simulink model "PVFCHEV_1"  (R2018a)
settings: Solver=VariableStepAuto  StartTime=0.0  StopTime=25  RelTol=1e-3
values from neighbouring files (symbols this model uses):
  Fc_current = [ 0  1.7  3.3  5.06  6.8   8.6  10.4   12.3  14.15   16   17.85  19.8   21.8   23.75   25.75   27.75  29.8  31.9  34.1  36.2  38.2  40.9  42.6  44.7   47.1   49.4   51.6    54   56.85  58.75  61.2  63.6  66.1  68.6  71.2  73.8 76.5 79.15  81.85  84.6  87.5   90.4  93.3      96.4   99.45  102.5    105.65   109   112.8  115.75  119.25   123     126.65     130.5      134.5   138.6  142.9 147.4  153.0 ...(+15 chars)    [pvfchev_configration.m]
  Fc_power = [ 0  100  200  300   400   500   600    700   800   900   1000   1100   1200   1300    1400    1500  1600   1700  1800  1900  2000  2100  2200  2300   2400   2500   2600   2700   2800  2900   3000  3100  3200 3300   3400  3500 3600 3700  3800   3900   4000   4100  4198.5    4300   4400   4500      4600   4700  4800    4900    5000    5100     5200       5300       5400    5500  5600  5700   5800   ...(+17 chars)    [pvfchev_configration.m]
  Ts_Control = 1e-04    (= 0.0001)    [pvfchev_configration.m]
  Ts_Power = 2e-06    [pvfchev_configration.m]
undefined symbols (not defined in the file or in its folder): DiscIntNeverNeededParam, Ion, Lithium
libraries: powerlib x30, powerlib_meascontrol x8, sdl_lib x8, fl_lib x6, nesl_utility x6, electricdrivelib x4, spsVIMeasurementModel x3, simulink x2, re_lib x1, spsDrivesPrivateModels x1, spsDrivesOutputSelector x1, spsDrivesSpeedControllerModel x1
(part 1 of 2)
settings Model: Creator=EUROPE LAPTOP  LastModifiedBy=Windows.10
settings SolverCC: AlgebraicLoopSolver=LineSearch
settings CodeAppCC: StateflowObjectComments=on
settings SimscapeCC: SimscapeNormalizeSystem=off

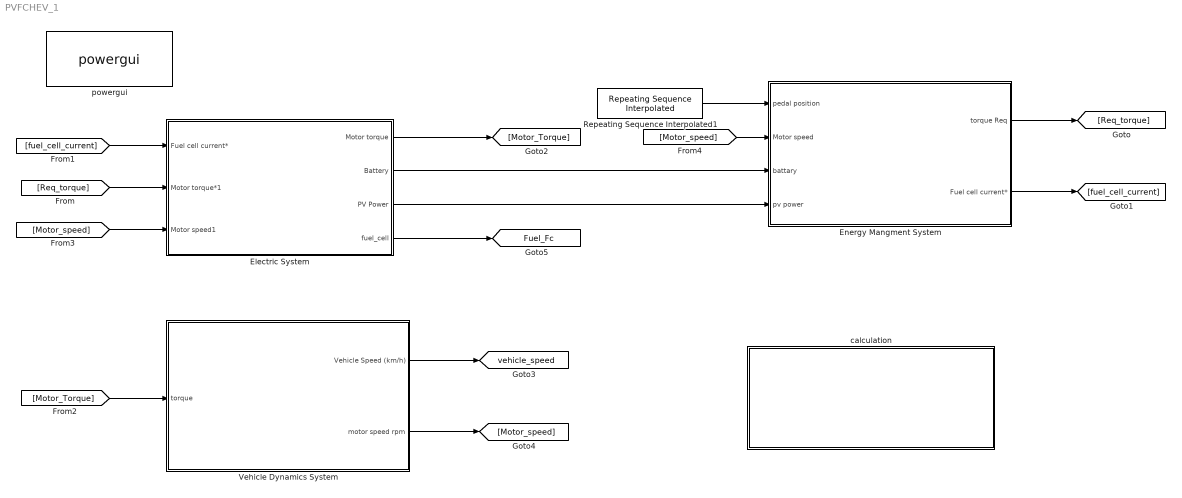
== system PVFCHEV_1 ==
  Electric System : Subsystem
  Energy Mangment System : Subsystem
  Repeating Sequence Interpolated1 : simulink/Sources/Repeating Sequence Interpolated  OutValues="[ 0 0 70 70 25 25  85  85 -70 -70].'"  TimeValues=[0 1.999 2 6 6.001 11 11.001 15.999 16 25].'  LookUpMeth=Interpolation-Use End Values  tsamp=0.01  OutMin=[]  OutMax=[]  OutDataTypeStr=double  OutputDataTypeScalingMode=double  OutDataType=fixdt(0,8)  OutScaling=2^-10
  Vehicle Dynamics System : Subsystem
  calculation : Subsystem
  powergui : powerlib/powergui  Priority=2  SimulationMode=Discrete  SampleTime=2e-6  frequency=60  Iterations=50  frequencyindice=0  Pbase=100e6  ErrMax=1e-4  UnitsV=kV  UnitsW=MW  buscounter=0  FunctionMessages=off  echomessages=off  EnableUseOfTLC=off  CurrentSourceSwitches=off  DisableSnubberDevices=off  DisableRonSwitches=off  DisableVfSwitches=off  DisplayEquations=off  SolverType=Tustin/Backward Euler (TBE)  Interpol=off  ExternalGateDelay=off  methode=off  Ts=100  x0status=blocks  SPID=off  SwTol=0  HookPort=off  RestoreLinks=warning  ResistiveCurrentMeasurement=off  Frange=[0:2:500]  Ylog=off  Xlog=on  ShowGrid=off  save=off  variable=ZData  structure=0  ZoomFFT=on  StartTime=0.0  cycles=1  DisplayStyle=1  fundamental=60  FreqAxis=off  MaxFrequency=1000  frequencyindicesteady=1  RmsSteady=1  display=off
  tag scope: Fuel_Fc=global, vehicle_speed=global
  wires:
  Energy Mangment System/2(Fuel cell current*) -> [fuel_cell_current]
  Electric System/1(Motor torque) -> [Motor_Torque]
  Electric System/3(PV Power) -> Energy Mangment System/4(pv power)
  [fuel_cell_current] -> Electric System/1("Fuel cell current* ")
  [Motor_Torque] -> Vehicle Dynamics System/1(torque)
  [Req_torque] -> Electric System/2(Motor torque*1)
  [Motor_speed] -> Energy Mangment System/2(Motor speed)
  Repeating Sequence Interpolated1/1 -> Energy Mangment System/1(pedal position)
  Energy Mangment System/1("torque Req ") -> [Req_torque]
  Vehicle Dynamics System/1(Vehicle Speed (km/h)) -> [vehicle_speed]
  Vehicle Dynamics System/2(motor speed rpm) -> [Motor_speed]
  [Motor_speed] -> Electric System/3(Motor speed1)
  Electric System/2(Battery) -> Energy Mangment System/3(battary)
  Electric System/4(fuel_cell) -> [Fuel_Fc]

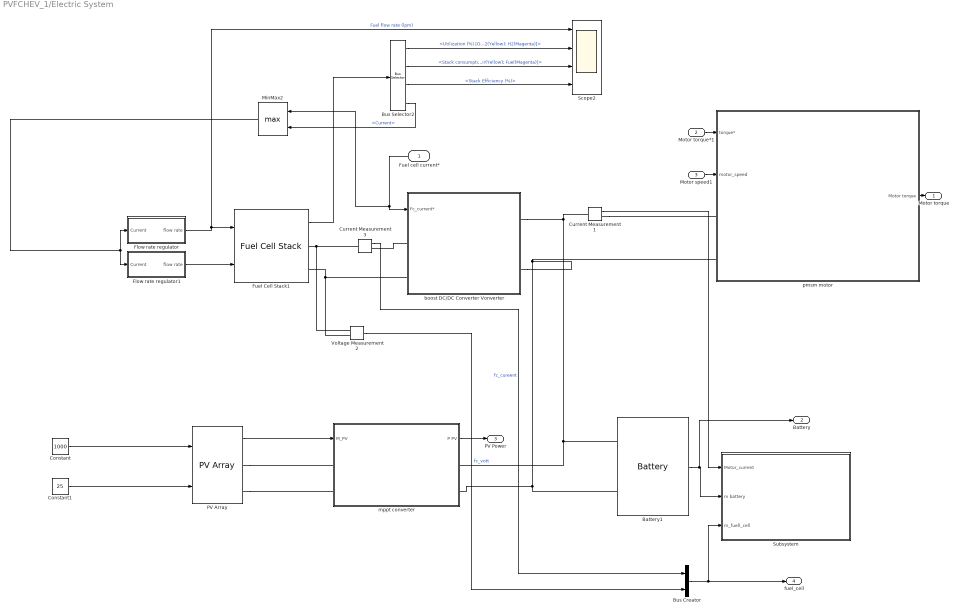
== system PVFCHEV_1/Electric System ==
  "Fuel cell current* " : Inport
  Motor torque*1 : Inport  Port=2
  Motor speed1 : Inport  Port=3
  Battery1 : electricdrivelib/Extra Sources/Battery  BatType=Lithium-Ion  ShowTempParam=off  ThermalPreset=no  ShowAgeParam=off  NomV=144  NomQ=9.6  SOC=74  Batt_Tr=30  PresetModel=on  MaxQ=9.6  MinV=108  FullV=167.6141  Dis_rate=4.1739  R=0.15  Normal_OP=8.6817  expZone="[155.5756     0.4716522]"  current=[6.5 13 32.5]  Units=Time  Tci=20  NomT=20  T2=-30  MaxQ2=4.8  FullV2=7.1  Normal_OP2=5.655  expZone2="[6.58           1]"  Rca=0.6  ti=2000  Dp=0  Neq0=0  Tsim=1e6  Ta1=25  Qeol=5.4*0.9  Reol=0.013333*1.2  Char_age=[2.3478, 3]  Dis_age=[2.3478, 10]  N1=1500  N2=10500  N3=1000  N4=1400  Ta2=45  N5=950
  Bus Creator : BusCreator  Inputs=2
  Bus Selector2 : BusSelector  OutputSignals=Utilization (%) [O2(Yellow); H2(Magenta)],Stack consumption (lpm) [Air(Yellow); Fuel(Magenta)],Stack Efficiency (%),Current
  Constant : Constant  Value=1000
  Constant1 : Constant  Value=25
  Current Measurement1 : powerlib/Measurements/Current Measurement  PhasorSimulation=off  OutputType=Complex  PSBequivalent=0
  Current Measurement3 : powerlib/Measurements/Current Measurement  PhasorSimulation=off  OutputType=Complex  PSBequivalent=0
  Flow rate regulator : Subsystem  mask{Nc=65, Uf_H2=99.56, T=65, Pf=1.5, x=99.95}
      mask prompts: Nc "Number of cells"; Uf_H2 "Nominal Hydrogen utilization (%)"; T "Operating temperature (Celsius)"; Pf "Fuel pressure (bar)"; x "H2 composition (%)"
  Flow rate regulator1 : Subsystem  mask{Nc=65, Uf_H2=99.56, T=65, Pf=1.5, x=99.95}
      mask prompts: Nc "Number of cells"; Uf_H2 "Nominal Hydrogen utilization (%)"; T "Operating temperature (Celsius)"; Pf "Fuel pressure (bar)"; x "H2 composition (%)"
  Fuel Cell Stack1 : electricdrivelib/Extra Sources/Fuel Cell Stack  PresetModel=No (User-Defined)  FcType=Proton Exchange Membrane (PEM)  Detailed=Detailed  Eoc="[65  63]"  NomVI="[93.3            45]"  EndVI="[162.16   37]"  Nc=65  n=55  TOp=65  AirFr=300  SuppPress="[1.5           1]"  Comp="[99.95           21            1]"  SignX=off  SignY=off  FlowRateH2=on  FlowRateAir=on  SystemTemp=off  SystemPH2=off  SystemPAir=off  FCDyn=off  FC_tau=0  Peak_O2=80  V_Under=10
      settings: SourceProductName=Simscape Power Systems  SourceProductBaseCode=PS
  MinMax2 : MinMax  Function=max  Inputs=2
  PV Array : re_lib/Solar/PV Array  Npar=1  Nser=2  PlotType=array @ 1000 W/m2 & specified temperatures  S_vec="[ 1000  500  100 ]"  Temp_C_vec="[  25  ]"  ModuleName=User-defined  PlotWhenSelected=off  Pm=249.952  Ncell=72  Voc=50.93  Isc=6.2  Vm=42.8  Im=5.84  beta_Voc_pc=-0.36099  alpha_Isc_pc=0.102  beta_Voc=-0.18385  alpha_Isc=0.006324  IL=6.2189  I0=2.3129e-10  nI=1.1472  Rsh=540.4905  Rs=0.29328  BAL=on  Tc=1e-6  Tfilter=5e-5
  Scope2 : Scope  NumInputPorts=4
  Subsystem : Subsystem
  Voltage Measurement2 : powerlib/Measurements/Voltage Measurement  PhasorSimulation=off  OutputType=Complex  PSBequivalent=0
  boost DC/DC Converter Vonverter : Subsystem
  mppt converter : Subsystem
  pmsm motor : Subsystem
      mask Display: image('C:\Users\Windows.10\Desktop\motor.png');
  Motor torque : Outport
  Battery : Outport  Port=2
  PV Power : Outport  Port=3
  fuel_cell : Outport  Port=4
  wires:
  pmsm motor/1(Motor torque) -> Motor torque/1
  Constant/1 -> PV Array/1
  Constant1/1 -> PV Array/2
  Bus Selector2/1 -> Scope2/2  "<Utilization (%) [O2(Yellow); H2(Magenta)]>"
  Bus Selector2/2 -> Scope2/3  "<Stack consumption (lpm) [Air(Yellow); Fuel(Magenta)]>"
  Fuel Cell Stack1/1 -> Bus Selector2/1
  Flow rate regulator/1(flow rate) -> Fuel Cell Stack1/1, Scope2/1  "Fuel flow rate (lpm)"
  MinMax2/1 -> Flow rate regulator/1(Current), Flow rate regulator1/1(Current)
  Flow rate regulator1/1(flow rate) -> Fuel Cell Stack1/2
  "Fuel cell current* "/1 -> MinMax2/1, boost DC/DC Converter Vonverter/1(Fc_current*)
  Current Measurement3/1 -> Bus Creator/1  "fc_cureent"
  Bus Selector2/3 -> Scope2/4  "<Stack Efficiency (%)>"
  Voltage Measurement2/1 -> Bus Creator/2  "fc_vott"
  Motor speed1/1 -> pmsm motor/2(motor_speed)
  Motor torque*1/1 -> pmsm motor/1(torque*)
  Battery1/1 -> Subsystem/2(m battery), Battery/1
  PV Array/1 -> mppt converter/1(M_PV)
  mppt converter/1(P PV) -> PV Power/1
  Bus Creator/1 -> Subsystem/3(m_fuell_cell), fuel_cell/1
  Current Measurement1/1 -> Subsystem/1(Motor_current)
  Bus Selector2/4 -> MinMax2/2  "<Current>"
  connections:
  PV Array/RConn1 -- mppt converter/LConn1
  PV Array/RConn2 -- mppt converter/LConn2
  Battery1/LConn1 -- mppt converter/RConn1 -- Current Measurement1/LConn1 -- boost DC/DC Converter Vonverter/RConn1
  Current Measurement3/LConn1 -- Voltage Measurement2/LConn1 -- Fuel Cell Stack1/RConn1
  boost DC/DC Converter Vonverter/LConn1 -- Current Measurement3/RConn1
  Voltage Measurement2/LConn2 -- Fuel Cell Stack1/RConn2 -- boost DC/DC Converter Vonverter/LConn2
  pmsm motor/LConn2 -- boost DC/DC Converter Vonverter/RConn2 -- mppt converter/RConn2 -- Battery1/LConn2
  Current Measurement1/RConn1 -- pmsm motor/LConn1

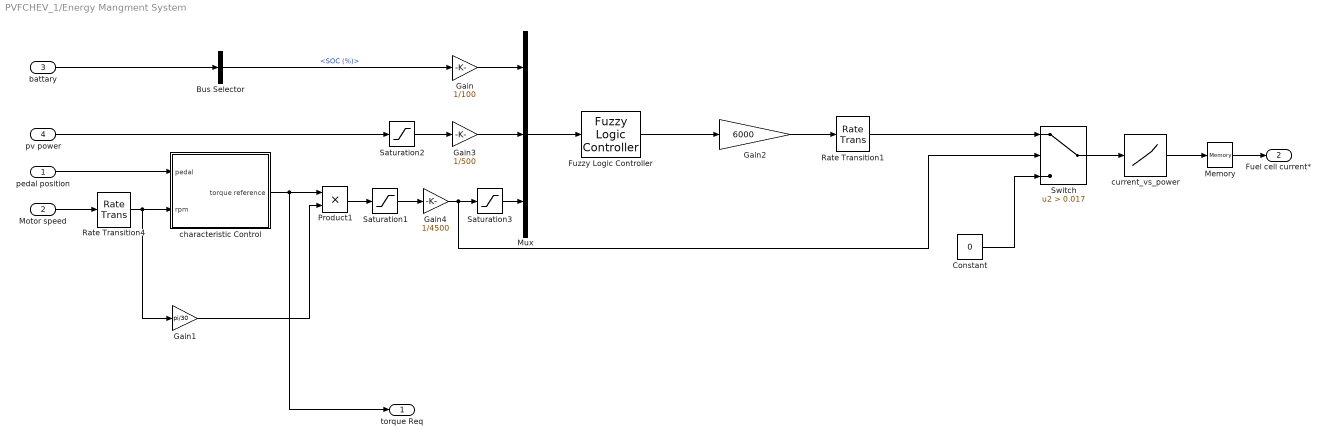
== system PVFCHEV_1/Energy Mangment System ==
  pedal position : Inport
  Motor speed : Inport  Port=2
  battary : Inport  Port=3
  pv power : Inport  Port=4
  Bus Selector : BusSelector  OutputSignals=SOC (%)
  Constant : Constant  Value=0
  Fuzzy Logic Controller : fuzblock/Fuzzy Logic  Controller  FIS=power_mangment  OutputSampleNumber=101  DataType=double  FuzzifiedInputs=off  RuleFiringStrengths=off  RuleOutputs=off  AggregatedOutputs=off  SimulateUsing=Interpreted execution  OutOfRangeInputValueMessage=warning  NoRuleFiredMessage=warning  EmptyOutputFuzzySetMessage=warning
  Gain : Gain  Gain=1/100
  Gain1 : Gain  Gain=pi/30
  Gain2 : Gain  Gain=6000
  Gain3 : Gain  Gain=1/500
  Gain4 : Gain  Gain=1/4500
  Memory : Memory  InitialCondition=0.00001
  Mux : Mux  Inputs=3
  Product1 : Product
  Rate Transition1 : RateTransition
  Rate Transition4 : RateTransition
  Saturation1 : Saturate  UpperLimit=4500  LowerLimit=-5000
  Saturation2 : Saturate  UpperLimit=500  LowerLimit=0
  Saturation3 : Saturate  UpperLimit=1  LowerLimit=0
  Switch : Switch  Criteria=u2 > Threshold  Threshold=0.017
  characteristic Control : Subsystem
  current_vs_power : Lookup  InputValues=Fc_power  Table=Fc_current
  "torque Req " : Outport
  Fuel cell current* : Outport  Port=2
  wires:
  battary/1 -> Bus Selector/1
  Bus Selector/1 -> Gain/1  "<SOC (%)>"
  pedal position/1 -> characteristic Control/1(pedal)
  Motor speed/1 -> Rate Transition4/1
  characteristic Control/1(torque reference) -> "torque Req "/1, Product1/1
  Mux/1 -> Fuzzy Logic Controller/1
  Fuzzy Logic Controller/1 -> Gain2/1
  Gain/1 -> Mux/1
  pv power/1 -> Saturation2/1
  Gain3/1 -> Mux/2
  Gain4/1 -> Saturation3/1, Switch/2
  Saturation2/1 -> Gain3/1
  Saturation1/1 -> Gain4/1
  current_vs_power/1 -> Memory/1
  Rate Transition4/1 -> Gain1/1, characteristic Control/2(rpm)
  Product1/1 -> Saturation1/1
  Gain2/1 -> Rate Transition1/1
  Constant/1 -> Switch/3
  Switch/1 -> current_vs_power/1
  Rate Transition1/1 -> Switch/1
  Memory/1 -> Fuel cell current*/1
  Gain1/1 -> Product1/2
  Saturation3/1 -> Mux/3

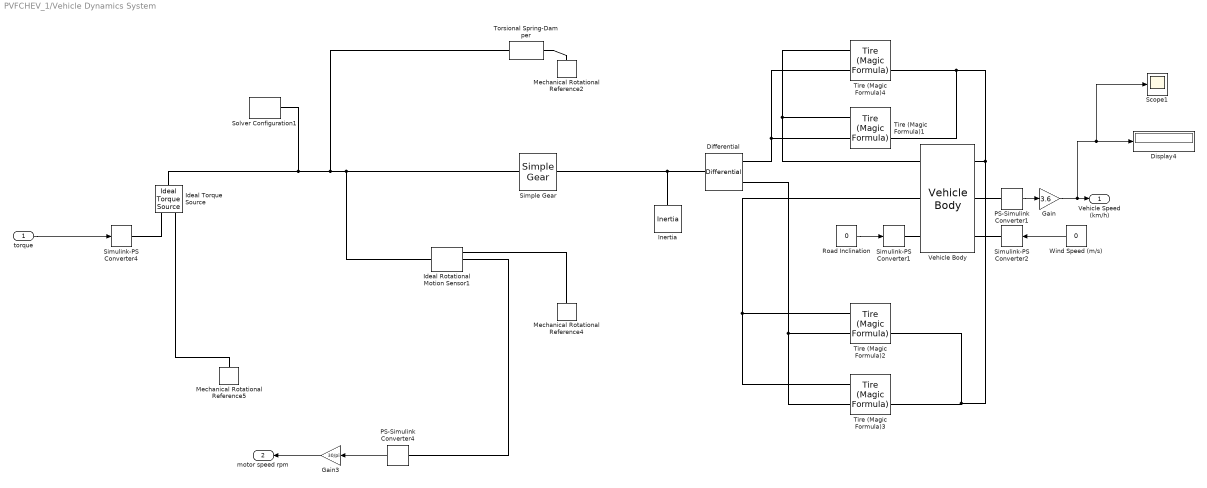
== system PVFCHEV_1/Vehicle Dynamics System ==
  torque : Inport
  Differential : sdl_lib/Gears/Differential  driveshaft_location=2  cd_ratio=1.2  friction_model=1  efficiency=[ 0.85 0.92 ]  mu_visc=[ 0 0 ] N*m/(rad/s)  pwr_thr=[ 0.001 0.001 ] W  carrier_inertia=0.001 kg*m^2  planet_inertia=0.0001 kg*m^2  temperature_TLU=[ 280 300 320 ] K  efficiency_ss_TLU=[ 0.95 0.9 0.85 ]  efficiency_cd_TLU=[ 0.95 0.9 0.85 ]  thermal_mass=50 J/K  T_init=300 K
      settings: SourceProductName=Simscape Driveline  SourceProductBaseCode=LD
  Display4 : Display
  Gain : Gain  Gain=3.6
  Gain3 : Gain  Gain=30/pi
  Ideal Rotational Motion Sensor1 : fl_lib/Mechanical/Mechanical Sensors/Ideal Rotational Motion Sensor  offset=0 rad
  Ideal Torque Source : fl_lib/Mechanical/Mechanical Sources/Ideal Torque Source
  Inertia : fl_lib/Mechanical/Rotational Elements/Inertia  inertia=0.0000001 kg*m^2  w_specify=off  w_priority=High  w=0 rad/s  w_nominal_specify=off  w_nominal_unit=rad/s  w_nominal_value=1  t_specify=off  t_priority=None  t=0 N*m  t_nominal_specify=off  t_nominal_unit=N*m  t_nominal_value=1
  Mechanical Rotational Reference2 : fl_lib/Mechanical/Rotational Elements/Mechanical Rotational Reference
  Mechanical Rotational Reference4 : fl_lib/Mechanical/Rotational Elements/Mechanical Rotational Reference
  Mechanical Rotational Reference5 : fl_lib/Mechanical/Rotational Elements/Mechanical Rotational Reference
  PS-Simulink Converter1 : nesl_utility/PS-Simulink Converter  PhysicalDomain=network_engine_domain  SubClassName=ps_output  LeftPortType=input  RightPortType=output  PseudoPeriodic=off  Frequencies=[]  Unit=m/s  AffineConversion=off
  PS-Simulink Converter4 : nesl_utility/PS-Simulink Converter  PhysicalDomain=network_engine_domain  SubClassName=ps_output  LeftPortType=input  RightPortType=output  PseudoPeriodic=off  Frequencies=[]  Unit=rad/s  AffineConversion=off
  Road Inclination : Constant  Value=0
  Scope1 : Scope
  Simple Gear : sdl_lib/Gears/Simple Gear  ratio=3  rotation_direction=1  friction_model=1  T_noload=0.1 N*m  T_nom=5 N*m  efficiency_nom=0.8  efficiency=0.8  mu_visc=[ 0 0 ] N*m/(rad/s)  w_thr=0.01 rad/s  pwr_thr=0.001 W  temperature_TLU=[ 280 300 320 ] K  load_TLU=[ 1 5 10 ] N*m  efficiency_TLU=[ 0.95 0.9 0.85 ]  efficiency_TLU2=[ 0.85 0.8 0.75; 0.95 0.9 0.85; 0.85 0.8 0.7 ]  thermal_mass=50 J/K  T_init=300 K
      settings: SourceProductName=Simscape Driveline
  Simulink-PS Converter1 : nesl_utility/Simulink-PS Converter  PhysicalDomain=network_engine_domain  SubClassName=ps_input  LeftPortType=input  RightPortType=output  PseudoPeriodic=off  Frequencies=[]  NoiseDistribution=none  NoiseParameters=[]  Unit=rad  AffineConversion=off  FilteringAndDerivatives=zero  SimscapeFilterOrder=1  InputFilterTimeConstant=.001  UdotUserProvided=1
  Simulink-PS Converter2 : nesl_utility/Simulink-PS Converter  PhysicalDomain=network_engine_domain  SubClassName=ps_input  LeftPortType=input  RightPortType=output  PseudoPeriodic=off  Frequencies=[]  NoiseDistribution=none  NoiseParameters=[]  Unit=m/s  AffineConversion=off  FilteringAndDerivatives=zero  SimscapeFilterOrder=1  InputFilterTimeConstant=.001  UdotUserProvided=1
  Simulink-PS Converter4 : nesl_utility/Simulink-PS Converter  PhysicalDomain=network_engine_domain  SubClassName=ps_input  LeftPortType=input  RightPortType=output  PseudoPeriodic=off  Frequencies=[]  NoiseDistribution=none  NoiseParameters=[]  Unit=N*m  AffineConversion=off  FilteringAndDerivatives=zero  SimscapeFilterOrder=1  InputFilterTimeConstant=.001  UdotUserProvided=1
  Solver Configuration1 : nesl_utility/Solver Configuration  PhysicalDomain=network_engine_domain  SubClassName=solver  LeftPortType=input  RightPortType=generic  Tones=[]  Harmonics=[]  SimulateNoise=off  Profile=off  UseLocalSampling=off  EnableSwitchedLinearOptims=on  FrequencyDomain=off  UseCCode=off  RelTol=0.001  AbsTol=1e-06  MinStep=1e-09  ToWorkspace=off  RevertToSquareIcSolve=off  NumHomotopyIterations=100  PhasorMode=off  PhasorModeNumHarmonics=1  DoDC=off  ResidualTolerance=1e-9  UseLocalSolver=on  LocalSolverChoice=NE_BACKWARD_EULER_ADVANCER  LocalSolverSampleTime=.001  DoFixedCost=on  MaxNonlinIter=3  MaxModeIter=2  LinearAlgebra=Sparse  EquationFormulation=NE_TIME_EF  DelaysMemoryBudget=1024  AutomaticFiltering=on  FilteringTimeConstant=0.001
  Tire (Magic Formula){1..4} (4 alike) : sdl_lib/Tires & Vehicles/Tire (Magic Formula)  parameterization=3  F_z1=1e+3 N  F_x1=3.5e+3 N  kappa1=10  B_m=10  C_m=1.9  D_m=1  E_m=0.97  fz0=4e+3 N  p_Cx=1.685  p_Dx=[ 1.21 -0.037 ]  p_Ex=[ 0.344 0.095 -0.02 0 ]  p_Kx=[ 21.51 -0.163 0.245 ]  p_Hx=[ -0.002 0.002 ]  p_Vx=[ 0 0 ]  v_tr_thr=0.1 m/s  r_e=0.2 m  model_compliance=0  stiffness=1e+6 N/m  damping=1000 N/(m/s)  model_inertia=0  inertia=1 kg*m^2  initial_velocity=0 rad/s  model_resistance=0  resistance_model=1  coeff=0.015  p_tire=250e3 Pa  alpha=-0.003  beta=0.97  coeff_a=84e-4  coeff_b=6.2e-4 s/m  coeff_c=1.6e-4 s^2/m^2  v_thr=1e-3 m/s
      settings: SourceProductName=Simscape Driveline
  Torsional Spring-Damper : sdl_lib/Couplings & Drives/Torsional Spring-Damper  k=0.0000005 N*m/rad  mu_visc=0.0000003 N*m/(rad/s)  trq_coulomb=0 N*m  static_kinetic_ratio=1.1  w_tol=0.001 rad/s  model_hardstop=0  upper_bound=10 deg  lower_bound=-10 deg  k_endstop=1e+6 N*m/rad  D_endstop=10 N*m/(rad/s)  hardstop_model=3  transition=0.001 rad  x0=0 deg
      settings: SourceProductName=Simscape Driveline  SourceProductBaseCode=LD
  Vehicle Body : sdl_lib/Tires & Vehicles/Vehicle Body  mass=800 kg  n_w=2  x_f=1 m  x_r=0.35 m  y_c=0.7 m  model_pitch=0  inertia=4000 kg*m^2  suspension_model=1  k_f=1e4 N/m  b_f=1e4 N/(m/s)  k_r=1e4 N/m  b_r=1e4 N/(m/s)  k_f_TLU=[-2000, -1000, 0, 1000, 2000] N  x_f_TLU=[-.4, -.2, 0, .2, .4] m  b_f_TLU=[-200, -100, 0, 100, 200] N  v_f_TLU=[-4, -2, 0, 2, 4] m/s  k_r_TLU=[-2000, -1000, 0, 1000, 2000] N  x_r_TLU=[-.4, -.2, 0, .2, .4] m  b_r_TLU=[-200, -100, 0, 100, 200] N  v_r_TLU=[-4, -2, 0, 2, 4] m/s  interp_method=simscape.enum.interpolation.linear  extrap_method=simscape.enum.extrapolation.linear  model_hardstop=0  upper_bound_f=.25 m  lower_bound_f=-.25 m  stop_k_f=1e6 N/m  stop_b_f=150 N/(m/s)  upper_bound_r=.25 m  lower_bound_r=-.25 m  stop_k_r=1e6 N/m  stop_b_r=150 N/(m/s)  initial_pitch=0 rad  initial_pitch_rate=0 rad/s  g=9.81 m/s^2  liftoff_warning=0  area=2.3 m^2  Cd=0.36  rho=1.18 kg/m^3  v_specify=on  v_priority=High  v=0 m/s  v_nominal_specify=off  v_nominal_unit=m/s  v_nominal_value=1
      settings: SourceProductName=Simscape Driveline
  Wind Speed (m/s) : Constant  Value=0
  Vehicle Speed (km/h) : Outport
  motor speed rpm : Outport  Port=2
  wires:
  Gain3/1 -> motor speed rpm/1
  torque/1 -> Simulink-PS Converter4/1
  PS-Simulink Converter1/1 -> Gain/1
  Wind Speed (m/s)/1 -> Simulink-PS Converter2/1
  Road Inclination/1 -> Simulink-PS Converter1/1
  PS-Simulink Converter4/1 -> Gain3/1
  Gain/1 -> Scope1/1, Display4/1, Vehicle Speed (km/h)/1
  connections:
  Tire (Magic Formula)2/LConn1 -- Vehicle Body/RConn2 -- Tire (Magic Formula)3/LConn1
  Tire (Magic Formula)2/RConn2 -- Vehicle Body/LConn1 -- Tire (Magic Formula)1/RConn2 -- Tire (Magic Formula)4/RConn2 -- Tire (Magic Formula)3/RConn2
  Tire (Magic Formula)2/LConn2 -- Tire (Magic Formula)3/LConn2 -- Differential/RConn1
  Tire (Magic Formula)1/LConn2 -- Tire (Magic Formula)4/LConn2 -- Differential/RConn2
  Tire (Magic Formula)4/LConn1 -- Vehicle Body/RConn1 -- Tire (Magic Formula)1/LConn1
  Differential/LConn1 -- Inertia/LConn1 -- Simple Gear/RConn1
  Mechanical Rotational Reference4/LConn1 -- Ideal Rotational Motion Sensor1/RConn1
  Simulink-PS Converter2/RConn1 -- Vehicle Body/LConn3
  Ideal Rotational Motion Sensor1/RConn2 -- PS-Simulink Converter4/LConn1
  Ideal Torque Source/LConn1 -- Solver Configuration1/RConn1 -- Torsional Spring-Damper/LConn1 -- Ideal Rotational Motion Sensor1/LConn1 -- Simple Gear/LConn1
  Torsional Spring-Damper/RConn1 -- Mechanical Rotational Reference2/LConn1
  Mechanical Rotational Reference5/LConn1 -- Ideal Torque Source/RConn2
  Simulink-PS Converter1/RConn1 -- Vehicle Body/RConn3
  PS-Simulink Converter1/LConn1 -- Vehicle Body/LConn2
  Simulink-PS Converter4/RConn1 -- Ideal Torque Source/RConn1

== system PVFCHEV_1/calculation ==
  Add2 : Sum  Inputs=+++-
  Mux2 : Mux  Inputs=6
  To File1 : ToFile  Filename=power.mat  MatrixName=power
  power_balance : Scope
  power_distrbution : Scope
  wires:
  [mot_power_Ts] -> Add2/4
  [bat_power_Ts] -> Add2/2
  [fc_power_out_Ts] -> Add2/1
  [pv_power_Ts] -> Add2/3
  Add2/1 -> power_balance/1
  [bat_power_Ts] -> Mux2/1  "bat"
  [fc_power_out_Ts] -> Mux2/2  "fc"
  [pv_power_Ts] -> Mux2/3  "pv"
  [mot_power_Ts] -> Mux2/4  "mot"
  [pv_power_source] -> Mux2/5  "pv_source"
  [fc_power_source] -> Mux2/6  "fc_source"
  Mux2/1 -> power_distrbution/1, To File1/1

== system PVFCHEV_1/Electric System/Flow rate regulator ==
  Current : Inport
  Fcn1 : Fcn  Expr=60000*8.3145*(273+T)*Nc*u(1)/(2*96485*(Pf*101325)*Uf_H2/100*x/100)
  Saturation : Saturate  UpperLimit=inf  LowerLimit=1
  flow rate : Outport
  wires:
  Fcn1/1 -> Saturation/1
  Current/1 -> Fcn1/1
  Saturation/1 -> flow rate/1

== system PVFCHEV_1/Electric System/Flow rate regulator1 ==
  Current : Inport
  Fcn1 : Fcn  Expr=60000*8.3145*(273+T)*65*u(1)/(4*96485*(0.9*101325)*0.5057*0.21)
  Saturation : Saturate  UpperLimit=inf  LowerLimit=1
  flow rate : Outport
  wires:
  Saturation/1 -> flow rate/1
  Current/1 -> Fcn1/1
  Fcn1/1 -> Saturation/1

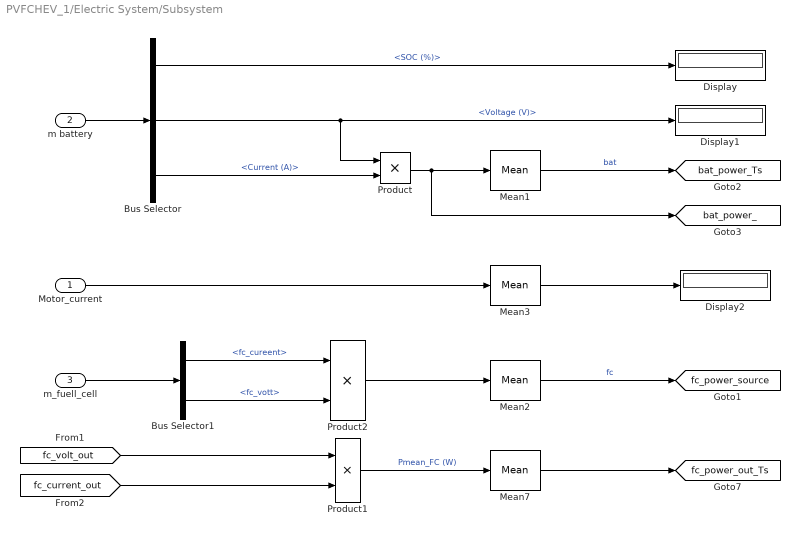
== system PVFCHEV_1/Electric System/Subsystem ==
  Motor_current : Inport
  m battery : Inport  Port=2
  m_fuell_cell : Inport  Port=3
  Bus Selector : BusSelector  OutputSignals=SOC (%),Voltage (V),Current (A)
  Bus Selector1 : BusSelector  OutputSignals=fc_cureent,fc_vott
  Display : Display
  Display1 : Display
  Display2 : Display
  Mean{1..3,7} (4 alike) : powerlib_meascontrol/Measurements/Mean  Freq=60  Vinit=0  Ts=Ts_Control
  Product : Product
  Product1 : Product  RndMeth=Zero
  Product2 : Product  RndMeth=Zero
  tag scope: bat_power_=global, bat_power_Ts=global, fc_power_out_Ts=global, fc_power_source=global
  wires:
  m battery/1 -> Bus Selector/1
  Bus Selector/1 -> Display/1  "<SOC (%)>"
  Bus Selector/2 -> Product/1, Display1/1  "<Voltage (V)>"
  Bus Selector/3 -> Product/2  "<Current (A)>"
  Motor_current/1 -> Mean3/1
  m_fuell_cell/1 -> Bus Selector1/1
  Product1/1 -> Mean7/1  "Pmean_FC (W)"
  Product/1 -> Mean1/1, [bat_power_]
  Bus Selector1/1 -> Product2/1  "<fc_cureent>"
  Bus Selector1/2 -> Product2/2  "<fc_vott>"
  [fc_volt_out] -> Product1/1
  [fc_current_out] -> Product1/2
  Mean1/1 -> [bat_power_Ts]  "bat"
  Product2/1 -> Mean2/1
  Mean2/1 -> [fc_power_source]  "fc"
  Mean3/1 -> Display2/1
  Mean7/1 -> [fc_power_out_Ts]

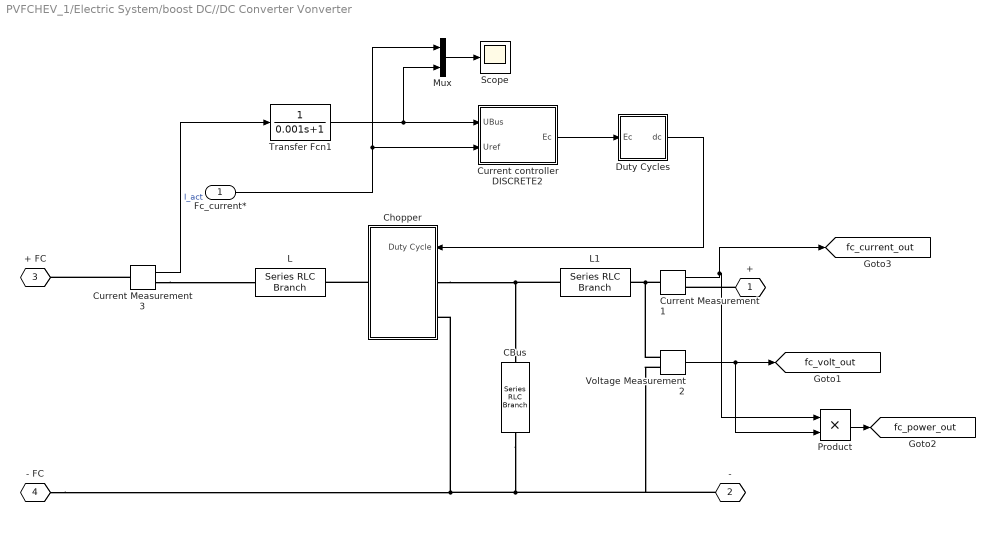
== system PVFCHEV_1/Electric System/boost DC//DC Converter Vonverter ==
  Fc_current* : Inport
  CBus : powerlib/Elements/Series RLC Branch  LConnTagsString=__new0  RConnTagsString=__new0  BranchType=RC  Resistance=0.2  Inductance=1e-3  SetiL0=off  InitialCurrent=0  Capacitance=7500e-6  Setx0=on  InitialVoltage=152  Measurements=None
  Chopper : Subsystem  mask(SPSdrives Converter){SnubberResistance=10e3, SnubberCapacitance=inf, Ron=1e-3, ForwardVoltages=[1.3,1.3], IGBTParameters=[0,0], converterType=Inverter}
      mask prompts: SnubberResistance "Snubber resistance Rs (Ohms):"; SnubberCapacitance "Snubber capacitance Cs (F):"; Ron "Ron (Ohms):"; ForwardVoltages "Forward voltages [Device Vf(V), Diode Vd (V)]"; IGBTParameters "[Tf(s), Tt(s)]:"; converterType "Converter type:"
      mask help: This model implements an average-value buck converter."Duty Cycle" contains the duty cycle of the internal IGBT device.
      mask TypeOptions converterType: Rectifier | Inverter
      mask Display: plot(0,0,100,100,[39 39 23.8],[71 28 28],[44 56 49.6 56 52.8 56 61 61],[39.2 33.6 32.8 33.6 40.8 33.6 30 12.4],[44 44 44 61 61],[28 71 60 66.4 90],[75 67 83 75 67 83 75 75],[54 42 42 54 54 54 54 66],[61 75 75],[24 24 42],[75 75 61],[66,76,76])
  Current Measurement1 : powerlib/Measurements/Current Measurement  PhasorSimulation=off  OutputType=Complex  PSBequivalent=0
  Current Measurement3 : powerlib/Measurements/Current Measurement  PhasorSimulation=off  OutputType=Complex  PSBequivalent=0
  Current controller DISCRETE2 : Subsystem  mask(PI controller){Kp=0.0005, Ki=0.15, Ts=1e-3}
      mask prompts: Kp "Proportional gain (Kp)"; Ki "Integral gain (Ki)"; Ts "Sample time (s) :"
      mask help: Proportional-Integral Speed Controller
      mask Display: plot(0,0,100,100,[35,35,65],[70,30,30],[35,65],[45,60])
  Duty Cycles : Subsystem
  L : powerlib/Elements/Series RLC Branch  LConnTagsString=__new0  RConnTagsString=__new0  BranchType=L  Resistance=0.3  Inductance=500e-6  SetiL0=on  InitialCurrent=5  Capacitance=100e-6  Setx0=off  InitialVoltage=0  Measurements=None
  L1 : powerlib/Elements/Series RLC Branch  LConnTagsString=__new0  RConnTagsString=__new0  BranchType=L  Resistance=0.3  Inductance=500e-6  SetiL0=on  InitialCurrent=0.0001  Capacitance=100e-6  Setx0=off  InitialVoltage=0  Measurements=None
  Mux : Mux  Inputs=2
  Product : Product
  Scope : Scope
  Transfer Fcn1 : TransferFcn  Denominator=[0.001 1]
  Voltage Measurement2 : powerlib/Measurements/Voltage Measurement  PhasorSimulation=off  OutputType=Complex  PSBequivalent=0
  + : PMIOPort  Tag=PMCPort  Side=Right
  - : PMIOPort  Tag=PMCPort  Port=2  Side=Right
  + FC : PMIOPort  Tag=PMCPort  Port=3  Side=Left
  - FC : PMIOPort  Tag=PMCPort  Port=4  Side=Left
  tag scope: fc_current_out=global, fc_power_out=global, fc_volt_out=global
  wires:
  Duty Cycles/1(dc) -> Chopper/1(Duty Cycle)
  Current controller DISCRETE2/1(Ec) -> Duty Cycles/1(Ec)
  Fc_current*/1 -> Mux/1, Current controller DISCRETE2/2(Uref)
  Mux/1 -> Scope/1
  Current Measurement3/1 -> Transfer Fcn1/1  "I_act"
  Transfer Fcn1/1 -> Mux/2, Current controller DISCRETE2/1(UBus)
  Voltage Measurement2/1 -> Product/2, [fc_volt_out]
  Current Measurement1/1 -> Product/1, [fc_current_out]
  Product/1 -> [fc_power_out]
  connections:
  - FC/RConn1 -- -/RConn1 -- Voltage Measurement2/LConn2 -- CBus/RConn1 -- Chopper/LConn2
  Chopper/LConn1 -- L1/RConn1 -- CBus/LConn1
  Chopper/RConn1 -- L/LConn1
  Current Measurement3/LConn1 -- + FC/RConn1
  Current Measurement3/RConn1 -- L/RConn1
  Current Measurement1/LConn1 -- Voltage Measurement2/LConn1 -- L1/LConn1
  +/RConn1 -- Current Measurement1/RConn1

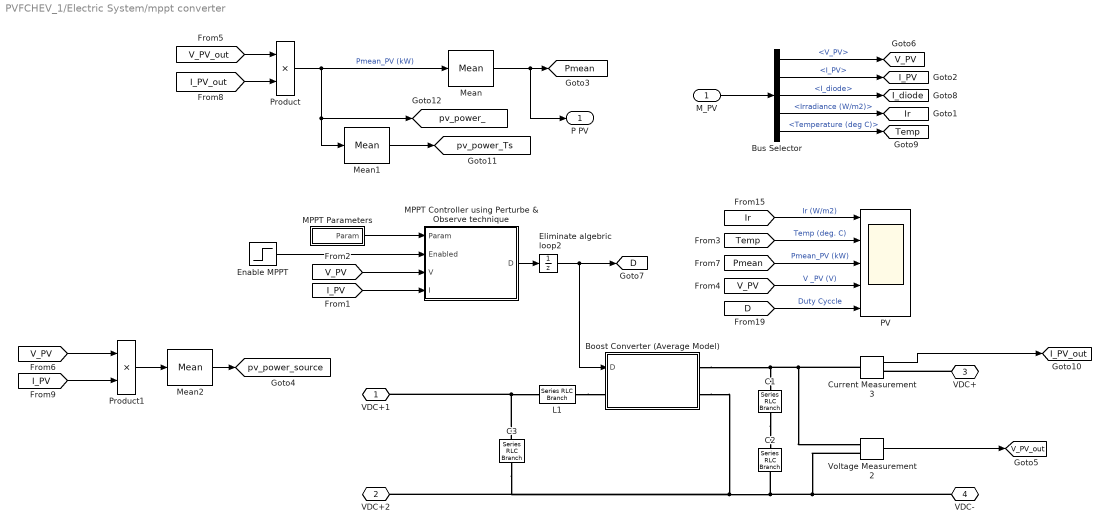
== system PVFCHEV_1/Electric System/mppt converter ==
  M_PV : Inport
  Boost Converter (Average Model) : Subsystem  mask(Boost Converter (Average Model)){Ts=Ts_Power}
      mask prompts: Ts "Sample time:"
      mask Display: disp('Boost\n(Average)')
  Bus Selector : BusSelector  OutputSignals=V_PV,I_PV,I_diode,Irradiance (W/m2),Temperature (deg C)
  C1 : powerlib/Elements/Series RLC Branch  LConnTagsString=__new0  RConnTagsString=__new0  BranchType=C  Resistance=1.0  Inductance=1.0  SetiL0=off  InitialCurrent=0  Capacitance=12000e-06  Setx0=off  InitialVoltage=0  Measurements=None
  C2 : powerlib/Elements/Series RLC Branch  LConnTagsString=__new0  RConnTagsString=__new0  BranchType=C  Resistance=1.0  Inductance=1.0  SetiL0=off  InitialCurrent=0  Capacitance=12000e-06  Setx0=off  InitialVoltage=0  Measurements=None
  C3 : powerlib/Elements/Series RLC Branch  LConnTagsString=__new0  RConnTagsString=__new0  BranchType=C  Resistance=1.0  Inductance=1.0  SetiL0=off  InitialCurrent=0  Capacitance=100e-6  Setx0=off  InitialVoltage=0  Measurements=Branch voltage
  Current Measurement3 : powerlib/Measurements/Current Measurement  PhasorSimulation=off  OutputType=Complex  PSBequivalent=0
  Eliminate algebric loop2 : UnitDelay  SampleTime=Ts_Control
  Enable MPPT : Step  Time=0.3  SampleTime=0
  L1 : powerlib/Elements/Series RLC Branch  LConnTagsString=__new0  RConnTagsString=__new0  BranchType=RL  Resistance=0.005  Inductance=5e-3  SetiL0=off  InitialCurrent=0  Capacitance=1e-6  Setx0=off  InitialVoltage=0  Measurements=None
  MPPT Parameters : Subsystem
  "MPPT Controller using Perturbe & Observe technique " : MATLAB Function  TreatAsAtomicUnit=on
  Mean : powerlib_meascontrol/Measurements/Mean  Freq=60  Vinit=0  Ts=0.001
  Mean1 : powerlib_meascontrol/Measurements/Mean  Freq=60  Vinit=0  Ts=Ts_Control
  Mean2 : powerlib_meascontrol/Measurements/Mean  Freq=60  Vinit=0  Ts=Ts_Control
  PV : Scope  NumInputPorts=5
  Product : Product  RndMeth=Zero
  Product1 : Product  RndMeth=Zero
  Voltage Measurement2 : powerlib/Measurements/Voltage Measurement  PhasorSimulation=off  OutputType=Complex  PSBequivalent=0
  VDC+1 : PMIOPort  Side=Left
  VDC+2 : PMIOPort  Port=2  Side=Left
  VDC+ : PMIOPort  Port=3  Side=Right
  VDC- : PMIOPort  Port=4  Side=Right
  P PV : Outport
  tag scope: D=global, I_PV=global, I_PV_out=global, I_diode=global, Ir=global, Pmean=global, Temp=global, V_PV=global, V_PV_out=global, pv_power_=global, pv_power_Ts=global, pv_power_source=global
  wires:
  MPPT Parameters/1(Param) -> "MPPT Controller using Perturbe & Observe technique "/1(Param)
  Bus Selector/3 -> [I_diode]  "<I_diode>"
  [V_PV] -> "MPPT Controller using Perturbe & Observe technique "/3(V)
  Eliminate algebric loop2/1 -> Boost Converter (Average Model)/1(D), [D]
  [Ir] -> PV/1  "Ir (W/m2)"
  [Pmean] -> PV/3  "Pmean_PV (kW)"
  [D] -> PV/5  "Duty Cyccle"
  Bus Selector/2 -> [I_PV]  "<I_PV>"
  [V_PV] -> PV/4  "V _PV (V)"
  Bus Selector/1 -> [V_PV]  "<V_PV>"
  [I_PV] -> "MPPT Controller using Perturbe & Observe technique "/4(I)
  Bus Selector/5 -> [Temp]  "<Temperature (deg C)>"
  Bus Selector/4 -> [Ir]  "<Irradiance (W/m2)>"
  Enable MPPT/1 -> "MPPT Controller using Perturbe & Observe technique "/2(Enabled)
  M_PV/1 -> Bus Selector/1
  "MPPT Controller using Perturbe & Observe technique "/1(D) -> Eliminate algebric loop2/1
  [Temp] -> PV/2  "Temp (deg. C)"
  [I_PV_out] -> Product/2
  Mean1/1 -> [pv_power_Ts]
  Mean/1 -> P PV/1, [Pmean]
  Product/1 -> [pv_power_], Mean1/1, Mean/1  "Pmean_PV (kW)"
  [V_PV_out] -> Product/1
  Product1/1 -> Mean2/1
  [V_PV] -> Product1/1
  Mean2/1 -> [pv_power_source]
  [I_PV] -> Product1/2
  Voltage Measurement2/1 -> [V_PV_out]
  Current Measurement3/1 -> [I_PV_out]
  connections:
  C3/LConn1 -- VDC+1/RConn1 -- L1/LConn1
  Voltage Measurement2/LConn2 -- C2/RConn1 -- C3/RConn1 -- VDC+2/RConn1 -- Boost Converter (Average Model)/RConn2 -- VDC-/RConn1
  Current Measurement3/LConn1 -- Boost Converter (Average Model)/RConn1 -- C1/LConn1 -- Voltage Measurement2/LConn1
  C1/RConn1 -- C2/LConn1
  L1/RConn1 -- Boost Converter (Average Model)/LConn1
  VDC+/RConn1 -- Current Measurement3/RConn1

== system PVFCHEV_1/Electric System/pmsm motor ==
  note: PM Synchronous 5kW, 15Nm, 3000rpm, Motor Drive (Ts=2e-6 s)
  torque* : Inport
  motor_speed : Inport  Port=2
  Gain2 : Gain  Gain=pi/30
  PM Synchronous Motor Drive1 : Subsystem  AncestorBlock=electricdrivelib/AC drives/PM Synchronous Motor Drive  DialogController=POWERSYS.PowerSysDialog  LoadFcn=|  mask(PM Synchronous Motor Drive){Rs=0.0171, Lls=0.0018, Lms=0.0018, MachineConstant=Flux linkage established by magnets (V.s), FluxCst=0.28, VoltageCst=126.966, TorqueCst=1.05, ia=0, ib=0, J=0.089, Friction=0.005, p=1, wm=0, thetam=0, Rsnb_rec=10e3, Csnb_rec=20e-9, Ron_rec=1e-3, Vf_rec=1.3, cap_bus=2000e-6, Rbrake=8, fbrake=4000, activationVoltage=120, shutdownVoltage=80, sourceFrequency=60, deviceType=IGBT / Diodes, Ron_inv=1e-3, Vf_inv=0.8, Vfd_inv=0.8, Tf=1e-6, Tt=2e-6, Tf_GTO=0, Tt_GTO=0, Rsnb_inv=5000, Csnb_inv=inf, regulationType=Torque regulation, Acc=1000, Dec=-1000, kp_sc=5, ki_sc=100, fc_sc=100, Tsc=7*20e-6, Tmin=-120, Tmax=80, modulationType=Hysteresis, h=0.1, kp_Id=200, ki_Id=1000, kp_Iq=200, ki_Iq=1000, fc_bus=50, car_freq=20000, freq_max=20e3, Tvect=20e-6, baseSampleTime=2e-06, outputBusMode=Multiple output buses, busLabels=off, MechanicalLoad=Speed w, modelDetailLevel=Detailed, driveType=AC6, AverageValue=off}
      | if ~isempty(get_param(gcb,'UserData')) 
      |       UserDataToSimulinkMask(gcbh,get_param(gcb,'driveType'));  
      |       set_param(gcb, 'UserData',[]);
      |       set_param(gcb,'UserDataPersistent','off');
      | end 
      | if strcmp(get_param(gcb,'AverageValue'),'on')
      |     set_param(gcb,'modelDetailLevel','Average');
      | end
      mask prompts: Rs "Resistance (ohm):"; Lls "D-axis inductance (H):"; Lms "Q-axis inductance (H):"; MachineConstant "Specify:"; ia "Phase A (A):"; ib "Phase B (A):"; J "Inertia (kg.m^2):"; Friction "Friction factor (N.m.s):"; p "Pole pairs:"; wm "Speed (rad/s):"; thetam "Angle (deg):"; Rsnb_rec "Resistance (ohm):"; Csnb_rec "Capacitance (F):"; Ron_rec "On-state resistance (ohm):"; Vf_rec "Forward voltage (V):"; cap_bus "Capacitance (F):"; Rbrake "Resistance (ohm):"; fbrake "Chopper frequency (Hz):"; activationVoltage "Activation voltage (V):"; shutdownVoltage "Shutdown voltage (V):"; sourceFrequency "Source frequency (Hz):"; deviceType "Device type:"; Ron_inv "On-state resistance (ohm):"; Vf_inv "Main device:"; Vfd_inv "Diode:"; Tf "Fall time (s):"; Tt "Tail time (s):"; Tf_GTO "Fall time (s):"; Tt_GTO "Tail time (s):"; Rsnb_inv "Resistance (ohm):"; Csnb_inv "Capacitance (F):"; regulationType "Regulation type:"; Acc "Acceleration:"; Dec "Deceleration:"; kp_sc "Proportional gain:"; ki_sc "Integral gain:"; fc_sc "Speed cutoff frequency (Hz):"; Tsc "Speed controller sampling time (s):"; Tmin "Negative:"; Tmax "Positive:"; modulationType "Modulation type:"; h "Current controller hysteresis bandwidth (A):"; kp_Id "Proportional gain:"; ki_Id "Integral gain:"; kp_Iq "Proportional gain:"; ki_Iq "Integral gain:"; fc_bus "DC bus voltage sensor cutoff frequency (Hz):"; car_freq "SVM switching frequency (Hz):"; freq_max "Maximum  switching frequency (Hz):"; Tvect "Controller sampling time (s):"; baseSampleTime "Base sample time:"; outputBusMode "Output bus mode:"; busLabels "Use bus labels"; MechanicalLoad "Mechanical input:"; modelDetailLevel "Model detail level:"; driveType "Drive type:"; AverageValue "Average value model"
      mask help: Implements a classical vector control drive for permanent synchronous motors.
      mask init:
      | [X1,X1m,X2,X2m,X3,X4,Y1,Y1m,Y2,Y2m,Y3,Y4,color1,color2,INp,OUTp,machineType,baseSampleTime] = spsDrivesMaskInit(gcb,driveType,AverageValue);
      settings: OpenFcn=sps_rtmsupport('OpenFcn',gcbh)
      mask Help: helpview(psbhelp)
      mask TypeOptions MachineConstant: Flux linkage established by magnets (V.s) | Voltage Constant (V_peak L-L / krpm) | Torque Constant (N.m / A_peak)
      mask Callback MachineConstant:
      | block = gcb;
      | MC = get_param(block,'MachineConstant');
      | set_param([block,'/','Permanent Magnet Synchronous Machine'],'MachineConstant',MC);
      | set_param([block,'/','VECT'],'MachineConstant',MC);
      | switch MC
      |     case 'Flux linkage established by magnets (V.s)'
      |         set_param([block,'/','Permanent Magnet Synchronous Machine'],'Flux',get_param(block,'FluxCst'))
      |     case 'Voltage Constant (V_peak L-L / krpm)'
      |         set_param([block,'/','Permanent Magnet Synchronous Machine'],'VoltageCst',get_param(block,'VoltageCst'))
      |     case 'Torque Constant (N.m / A_peak)'
      |         set_param([block,'/','Permanent Magnet Synchronous Machine'],'TorqueCst',get_param(block,'TorqueCst'))
      | end
      mask Callback FluxCst:
      | block = gcb;
      | MC = get_param(block,'MachineConstant');
      | set_param([block,'/','Permanent Magnet Synchronous Machine'],'MachineConstant',MC);
      | set_param([block,'/','VECT'],'MachineConstant',MC);
      | switch MC
      |     case 'Flux linkage established by magnets (V.s)'
      |         set_param([block,'/','Permanent Magnet Synchronous Machine'],'Flux',get_param(block,'FluxCst'))
      |     case 'Voltage Constant (V_peak L-L / krpm)'
      |         set_param([block,'/','Permanent Magnet Synchronous Machine'],'VoltageCst',get_param(block,'VoltageCst'))
      |     case 'Torque Constant (N.m / A_peak)'
      |         set_param([block,'/','Permanent Magnet Synchronous Machine'],'TorqueCst',get_param(block,'TorqueCst'))
      | end
      mask Callback VoltageCst:
      | block = gcb;
      | MC = get_param(block,'MachineConstant');
      | set_param([block,'/','Permanent Magnet Synchronous Machine'],'MachineConstant',MC);
      | set_param([block,'/','VECT'],'MachineConstant',MC);
      | switch MC
      |     case 'Flux linkage established by magnets (V.s)'
      |         set_param([block,'/','Permanent Magnet Synchronous Machine'],'Flux',get_param(block,'FluxCst'))
      |     case 'Voltage Constant (V_peak L-L / krpm)'
      |         set_param([block,'/','Permanent Magnet Synchronous Machine'],'VoltageCst',get_param(block,'VoltageCst'))
      |     case 'Torque Constant (N.m / A_peak)'
      |         set_param([block,'/','Permanent Magnet Synchronous Machine'],'TorqueCst',get_param(block,'TorqueCst'))
      | end
      mask Callback TorqueCst:
      | block = gcb;
      | MC = get_param(block,'MachineConstant');
      | set_param([block,'/','Permanent Magnet Synchronous Machine'],'MachineConstant',MC);
      | set_param([block,'/','VECT'],'MachineConstant',MC);
      | switch MC
      |     case 'Flux linkage established by magnets (V.s)'
      |         set_param([block,'/','Permanent Magnet Synchronous Machine'],'Flux',get_param(block,'FluxCst'))
      |     case 'Voltage Constant (V_peak L-L / krpm)'
      |         set_param([block,'/','Permanent Magnet Synchronous Machine'],'VoltageCst',get_param(block,'VoltageCst'))
      |     case 'Torque Constant (N.m / A_peak)'
      |         set_param([block,'/','Permanent Magnet Synchronous Machine'],'TorqueCst',get_param(block,'TorqueCst'))
      | end
      mask TypeOptions deviceType: GTO / Diodes | MOSFET / Diodes | IGBT / Diodes
      mask Callback deviceType: set_param([gcb,'/Three-phase Inverter'],'Device',get_param(gcb,'deviceType'));
      mask TypeOptions regulationType: Speed regulation | Torque regulation
      mask Callback regulationType: set_param([gcb '/Speed Controller'],'SwK',get_param(gcb,'regulationType'));
      mask TypeOptions modulationType: Hysteresis | SVM
      mask TypeOptions outputBusMode: Multiple output buses | Single output bus
      mask TypeOptions MechanicalLoad: Torque Tm | Speed w | Mechanical rotational port
      mask TypeOptions modelDetailLevel: Detailed | Average
      mask Callback modelDetailLevel:
      | if strcmp(get_param(gcb,'modelDetailLevel'),'Average')
      |    set_param(gcb,'AverageValue','on');
      | else
      |    set_param(gcb,'AverageValue','off');
      | end
      mask TypeOptions driveType: AC6
      mask DialogControl Container7 Prompt: Permanent Magnet Synchronous Machine
      mask DialogControl Container22 Prompt: Electrical parameters
      mask DialogControl Container27 Prompt: Equivalent circuit parameters
      mask DialogControl Container21 Prompt: Flux constant
      mask DialogControl Container34 Prompt: Initial currents
      mask DialogControl Container23 Prompt: Mechanical parameters
      mask DialogControl Container36 Prompt: Initial  values
      mask DialogControl Container10 Prompt: Converters and DC bus
      mask DialogControl Container28 Prompt: Rectifier
      mask DialogControl Container26 Prompt: Snubbers
      mask DialogControl Container29 Prompt: Diodes
      mask DialogControl Container30 Prompt: DC bus
      mask DialogControl Container31 Prompt: Braking chopper
      mask DialogControl Container32 Prompt: Inverter
      mask DialogControl Container37 Prompt: Switches
      mask DialogControl Forwardvoltages Prompt: Forward voltages (V)
      mask DialogControl Turnoff Prompt: Turn-off characteristics
      mask DialogControl InvSnubbers Prompt: Snubbers
      mask DialogControl Container12 Prompt: Controller
      mask DialogControl Control5 Prompt: Schematic
      mask DialogControl Control5 Callback:
      | openfig('ac6.fig','invisible');
      | movegui(gcf,'northwest');
      | set(gcf,'Visible','on');
      mask DialogControl Container33 Prompt: Speed controller
      mask DialogControl Speedramp Prompt: Speed ramps (rpm/s)
      mask DialogControl PIregulator Prompt: PI regulator
      mask DialogControl Container43 Prompt: Torque output limits (N.m)
      mask DialogControl Container35 Prompt: Vector control
      mask DialogControl d_axiscurrentregulator Prompt: d-axis current regulator
      mask DialogControl q_axiscurrentregulator Prompt: q-axis current regulator
      mask DialogControl Container47 Prompt: Parameters file options
      mask DialogControl Control3 Prompt: Load
      mask DialogControl Control3 Callback: loadValues(gcb,get_param(gcb,'driveType'));
      mask DialogControl Control4 Prompt: Save
      mask DialogControl Control4 Callback: saveValues(gcb,get_param(gcb,'driveType'));
      mask Display:
      | patch([X1 X1m],[Y1 Y1m],color1);
      | patch(X3,Y3,color2);
      | plot([X1 X1m X2 X2m X3 X4],[Y1 Y1m Y2 Y2m Y3 Y4]);
      | text(0.5,0.3,'AC6','HorizontalAlignment','center')
      | HaveSPSMec = (strcmp(MechanicalLoad,'Torque Tm') || strcmp(MechanicalLoad,'Speed w'));
      | color('blue');
      | if (HaveSPSMec==1 && strcmp(outputBusMode,'Multiple output buses'))
      |     port_label('input',2,INp)
      |     port_label('output',4,OUTp)
      | end
      | if (HaveSPSMec==1 && strcmp(outputBusMode,'Single output bus'))
      |     port_label('input',2,INp)
      |     port_label('output',2,OUTp)
      | end
  PMSM Drive : Scope  NumInputPorts=5
  Rate Transition1 : RateTransition
  demux : Subsystem
  VDC+ : PMIOPort  Side=Left
  VDC- : PMIOPort  Port=2  Side=Left
  Motor torque : Outport
  tag scope: Motor_power=global
  wires:
  demux/2(speed) -> PMSM Drive/2  "Rotor speed (rpm)"
  Rate Transition1/1 -> PM Synchronous Motor Drive1/1(SP)
  demux/4(Current) -> PMSM Drive/4  "Current (I, Iq, Id)"
  PM Synchronous Motor Drive1/2(Conv.) -> [Motor_power]
  Gain2/1 -> PM Synchronous Motor Drive1/2(Tm)
  demux/1(Torque) -> PMSM Drive/1  "Electromagnetic Torque (Nm)  [measured, reference]"
  motor_speed/1 -> Gain2/1
  PM Synchronous Motor Drive1/3(Ctrl) -> demux/2(Ctrl)
  demux/5(Voltage) -> PMSM Drive/5  "Voltage (V, Vq, Vd)"
  torque*/1 -> Rate Transition1/1
  demux/3(Power) -> PMSM Drive/3  "Mechanical power (W)  [measured, reference]"
  PM Synchronous Motor Drive1/4(Wm) -> Motor torque/1
  PM Synchronous Motor Drive1/1(Motor) -> demux/1(motor)
  connections:
  PM Synchronous Motor Drive1/LConn2 -- VDC-/RConn1
  PM Synchronous Motor Drive1/LConn1 -- VDC+/RConn1

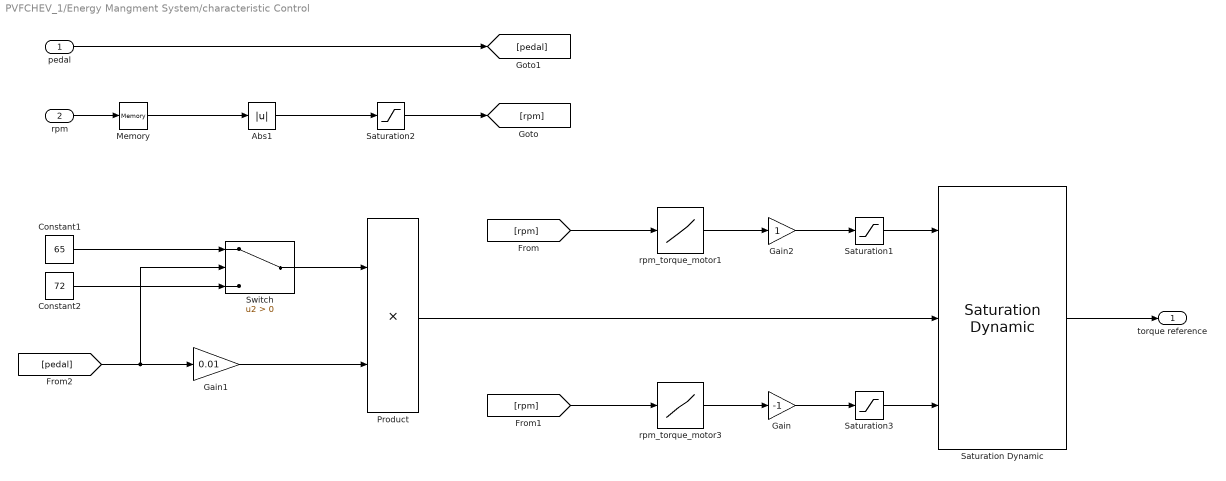
== system PVFCHEV_1/Energy Mangment System/characteristic Control ==
  pedal : Inport
  rpm : Inport  Port=2
  Abs1 : Abs
  Constant1 : Constant  Value=65
  Constant2 : Constant  Value=72
  Gain : Gain  Gain=-1
  Gain1 : Gain  Gain=0.01
  Gain2 : Gain
  Memory : Memory
  Product : Product
  Saturation Dynamic : simulink/Discontinuities/Saturation Dynamic  OutMin=[]  OutMax=[]  OutDataTypeStr=Inherit: Same as second input  OutDataType=fixdt(1, 16)  OutScaling=2^-10  DoSatur=off
  Saturation1 : Saturate  UpperLimit=50  LowerLimit=0
  Saturation2 : Saturate  UpperLimit=3000  LowerLimit=0
  Saturation3 : Saturate  UpperLimit=0  LowerLimit=-50
  Switch : Switch  Criteria=u2 > Threshold
  rpm_torque_motor1 : Lookup  InputValues="[0 500  900 1300  1700  2200  2600 3000]"  Table="[50  50  50  34.5  26.4   20.5 17  15]"  RndMeth=Ceiling
  rpm_torque_motor3 : Lookup  InputValues="[0 500  1000 1500  2000  2500  3000]"  Table="[50  50  50  34   25  20.5 17]"  RndMeth=Ceiling
  torque reference : Outport
  wires:
  [rpm] -> rpm_torque_motor1/1
  Product/1 -> Saturation Dynamic/2
  Saturation Dynamic/1 -> torque reference/1
  Gain1/1 -> Product/2
  rpm_torque_motor3/1 -> Gain/1
  [rpm] -> rpm_torque_motor3/1
  rpm/1 -> Memory/1
  Abs1/1 -> Saturation2/1
  pedal/1 -> [pedal]
  [pedal] -> Switch/2, Gain1/1
  Saturation2/1 -> [rpm]
  Memory/1 -> Abs1/1
  Constant1/1 -> Switch/1
  Constant2/1 -> Switch/3
  Switch/1 -> Product/1
  Saturation1/1 -> Saturation Dynamic/1
  Saturation3/1 -> Saturation Dynamic/3
  rpm_torque_motor1/1 -> Gain2/1
  Gain/1 -> Saturation3/1
  Gain2/1 -> Saturation1/1

== system PVFCHEV_1/Electric System/boost DC//DC Converter Vonverter/Chopper ==
  Duty Cycle : Inport
  Average-value armature voltage : Fcn  Expr=u(1)*u(2)
  Average-value source current : Fcn  Expr=u(1)*u(2)
  Bus to Vector : BusToVector
  Controlled Current Source : powerlib/Electrical Sources/Controlled Current Source  Initialize=on  Source_Type=AC  Amplitude=0  Phase=0  Frequency=0  Measurements=None
  Controlled Voltage Source : powerlib/Electrical Sources/Controlled Voltage Source  Initialize=on  Source_Type=AC  Amplitude=0  Phase=0  Frequency=0  Measurements=None
  Current Measurement : powerlib/Measurements/Current Measurement  Tag=PoWeRsYsTeMmEaSuReMeNt  PhasorSimulation=off  OutputType=Magnitude  PSBequivalent=0
  Memory : Memory
  Memory1 : Memory
  Mux : Mux  Inputs=2
  Mux1 : Mux  Inputs=2
  Selector : Selector  InputPortWidth=2  IndexOptions=Index vector (dialog)  Indices=[1]  OutputSizes=1
  Voltage Measurement1 : powerlib/Measurements/Voltage Measurement  Tag=PoWeRsYsTeMmEaSuReMeNt  PhasorSimulation=off  OutputType=Magnitude  PSBequivalent=0
  A : PMIOPort  Side=Right
  + : PMIOPort  Port=2  Side=Left
  - : PMIOPort  Port=3  Side=Left
  wires:
  Selector/1 -> Mux1/1, Mux/1
  Memory1/1 -> Controlled Current Source/1
  Average-value source current/1 -> Memory1/1
  Current Measurement/1 -> Mux1/2
  Mux1/1 -> Average-value source current/1
  Duty Cycle/1 -> Bus to Vector/1
  Voltage Measurement1/1 -> Mux/2
  Mux/1 -> Average-value armature voltage/1
  Average-value armature voltage/1 -> Memory/1
  Memory/1 -> Controlled Voltage Source/1
  Bus to Vector/1 -> Selector/1
  connections:
  A/RConn1 -- Current Measurement/RConn1
  Controlled Voltage Source/RConn1 -- Current Measurement/LConn1
  +/RConn1 -- Voltage Measurement1/LConn1 -- Controlled Current Source/LConn1
  Controlled Voltage Source/LConn1 -- -/RConn1 -- Controlled Current Source/RConn1 -- Voltage Measurement1/LConn2

== system PVFCHEV_1/Electric System/boost DC//DC Converter Vonverter/Current controller DISCRETE2 ==
  UBus : Inport
  Uref : Inport  Port=2
  Ctrl sat. : Saturate  UpperLimit=0.95  LowerLimit=-0.95
  Discrete-Time Integrator : DiscreteIntegrator  IntegratorMethod=Integration: Trapezoidal  SampleTime=Ts  LimitOutput=on  UpperSaturationLimit=0.95  LowerSaturationLimit=-0.95  ICPrevOutput=DiscIntNeverNeededParam  ICPrevScaledInput=DiscIntNeverNeededParam
  Integral gain : Gain  Gain=Ki  SaturateOnIntegerOverflow=on  OutDataTypeStr=Inherit: Same as input  ParamDataTypeStr=Inherit: Same as input
  Proportional gain : Gain  Gain=Kp  SaturateOnIntegerOverflow=on  OutDataTypeStr=Inherit: Same as input  ParamDataTypeStr=Inherit: Same as input
  Sum1 : Sum  Inputs=+-  SaturateOnIntegerOverflow=on  InputSameDT=on  OutDataTypeStr=Inherit: Same as first input
  Sum2 : Sum  SaturateOnIntegerOverflow=on  InputSameDT=on  OutDataTypeStr=Inherit: Same as first input
  Ec : Outport  InitialOutput=0
  wires:
  Proportional gain/1 -> Sum2/1
  Integral gain/1 -> Discrete-Time Integrator/1
  Sum1/1 -> Integral gain/1, Proportional gain/1
  UBus/1 -> Sum1/1
  Uref/1 -> Sum1/2
  Discrete-Time Integrator/1 -> Sum2/2
  Sum2/1 -> Ctrl sat./1
  Ctrl sat./1 -> Ec/1

== system PVFCHEV_1/Electric System/boost DC//DC Converter Vonverter/Duty Cycles ==
  Ec : Inport
  Add : Sum  Inputs=+-
  Bus Creator2 : BusCreator  Inputs=2
  Constant : Constant
  Duty Cycle : Fcn  Expr=0.5*(u[1]+1)
  dc : Outport
  wires:
  Bus Creator2/1 -> dc/1
  Ec/1 -> Duty Cycle/1
  Constant/1 -> Add/1
  Add/1 -> Bus Creator2/2  "IGBT 2"
  Duty Cycle/1 -> Bus Creator2/1, Add/2  "IGBT I"

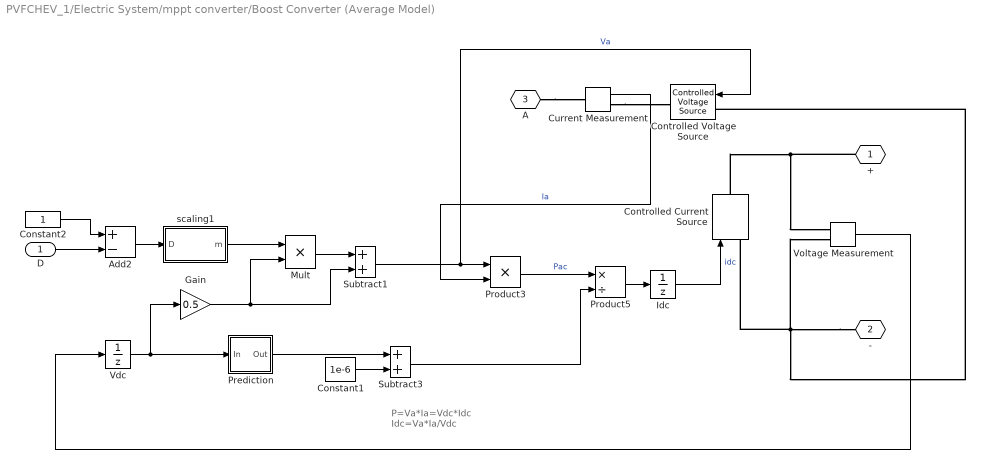
== system PVFCHEV_1/Electric System/mppt converter/Boost Converter (Average Model) ==
  note: P=Va*Ia=Vdc*Idc
      | Idc=Va*Ia/Vdc
  D : Inport
  Add2 : Sum  Inputs=+-
  Constant1 : Constant  Value=1e-6
  Constant2 : Constant
  Controlled Current Source : powerlib/Electrical Sources/Controlled Current Source  Initialize=on  Source_Type=AC  Amplitude=0  Phase=0  Frequency=0  Measurements=None
  Controlled Voltage Source : powerlib/Electrical Sources/Controlled Voltage Source  Initialize=on  Source_Type=AC  Amplitude=0  Phase=0  Frequency=0  Measurements=None
  Current Measurement : powerlib/Measurements/Current Measurement  PhasorSimulation=off  OutputType=Complex  PSBequivalent=0
  Gain : Gain  Gain=0.5
  Idc : UnitDelay  SampleTime=Ts
  Mult : Product  Inputs=**
  Prediction : Subsystem
  Product3 : Product  RndMeth=Zero
  Product5 : Product  Inputs=*/  RndMeth=Zero
  Subtract1 : Sum
  Subtract3 : Sum
  Vdc : UnitDelay  SampleTime=Ts
  Voltage Measurement : powerlib/Measurements/Voltage Measurement  PhasorSimulation=off  OutputType=Complex  PSBequivalent=0
  scaling1 : Subsystem
  + : PMIOPort  Tag=PMCPort  Side=Right
  - : PMIOPort  Tag=PMCPort  Port=2  Side=Right
  A : PMIOPort  Tag=PMCPort  Port=3  Side=Left
  wires:
  Gain/1 -> Mult/2, Subtract1/2
  Product5/1 -> Idc/1
  Constant1/1 -> Subtract3/2
  Subtract3/1 -> Product5/2
  Product3/1 -> Product5/1  "Pac"
  Prediction/1(Out) -> Subtract3/1
  Vdc/1 -> Prediction/1(In), Gain/1
  Subtract1/1 -> Product3/1, Controlled Voltage Source/1  "Va"
  Mult/1 -> Subtract1/1
  Constant2/1 -> Add2/1
  Add2/1 -> scaling1/1(D)
  scaling1/1(m) -> Mult/1
  D/1 -> Add2/2
  Voltage Measurement/1 -> Vdc/1
  Idc/1 -> Controlled Current Source/1  "idc"
  Current Measurement/1 -> Product3/2  "Ia"
  connections:
  -/RConn1 -- Voltage Measurement/LConn2 -- Controlled Voltage Source/LConn1 -- Controlled Current Source/LConn1
  +/RConn1 -- Voltage Measurement/LConn1 -- Controlled Current Source/RConn1
  Current Measurement/RConn1 -- Controlled Voltage Source/RConn1
  A/RConn1 -- Current Measurement/LConn1

== system PVFCHEV_1/Electric System/mppt converter/MPPT Parameters ==
  note: Upper limit for D (Dmax)
  note: Increment value used to increase/decrease (DeltaD)
  note: Initial value for D output (Dinit)
  note: (D = Boost converter duty cycle)
  note: Lower limit for D (Dmax)
  note: Parameters for Perturb and Observe Algorithm:
  Iph_ : Constant  Value=0.5
  Iph_1 : Constant  Value=0.58
  Iph_2 : Constant  Value=0.38
  Iph_3 : Constant  Value=3e-4
  Mux : Mux
  Param : Outport
  wires:
  Iph_/1 -> Mux/1
  Iph_1/1 -> Mux/2
  Iph_2/1 -> Mux/3
  Iph_3/1 -> Mux/4
  Mux/1 -> Param/1
